simulink model "quadrotor_dynamics_model"  (R2024b)
settings: Solver=VariableStepAuto  StartTime=0.0  FixedStep=0.001  RelTol=1e-3
values from neighbouring files (symbols this model uses):
  a_x_max = 5    [parameters.m]
  a_y_max = 5    [parameters.m]
  a_z_max = 5    [parameters.m]
  angle_max = 0.1745    [parameters.m]
  g = 9.81    [parameters.m]
  Ixx = 5e-3    (= 0.005)    [parameters.m]
  Iyy = 5e-3    (= 0.005)    [parameters.m]
  Izz = 1e-2    (= 0.01)    [parameters.m]
  Jr = 3e-5    (= 3e-05)    [parameters.m]
  K_d_x = 1e-7    (= 1e-07)    [parameters.m]
  K_d_y = 1e-7    (= 1e-07)    [parameters.m]
  K_d_z = 1e-7    (= 1e-07)    [parameters.m]
  Kd = 1e-7    (= 1e-07)    [parameters.m]
  Kd_pqr = [0, 0, 0]    [parameters.m]
  Kd_v = [0, 0, 0]    [parameters.m]
  Ki_pqr = [0.1, 0.1, 0.1]    [parameters.m]
  Ki_v = [0.1, 0.1, 0.1]    [parameters.m]
  Kp_phi = 12    [parameters.m]
  Kp_pqr = [2, 2, 2]    [parameters.m]
  Kp_psi = 10    [parameters.m]
  Kp_theta = 12    [parameters.m]
  Kp_v = [1, 1, 1]    [parameters.m]
  Kp_x = 0.1    [parameters.m]
  Kp_y = 0.1    [parameters.m]
  Kp_z = 0.1    [parameters.m]
  Kt = 3e-6    (= 3e-06)    [parameters.m]
  l = 0.2    [parameters.m]
  m = 0.5    [parameters.m]
  omega_sq_max = 5e+6    (= 5000000)    [parameters.m]
  p_max = 1    [parameters.m]
  q_max = 1    [parameters.m]
  r_max = 1    [parameters.m]
  rpy_dot_in = [0, 0, 0]    [parameters.m]
  rpy_in = [0, 0, 0]    [parameters.m]
  tau_x_max = 0.5    [parameters.m]
  tau_y_max = 0.5    [parameters.m]
  tau_z_max = 0.5    [parameters.m]
  v_x_max = 10    [parameters.m]
  v_y_max = 10    [parameters.m]
  v_z_max = 10    [parameters.m]
  xyz_dot_in = [0, 0, 0]    [parameters.m]
  xyz_in = [0, 0, 0]    [parameters.m]
libraries: slpidlib x6
settings Model: Creator=Ishan  LastModifiedBy=Ishan

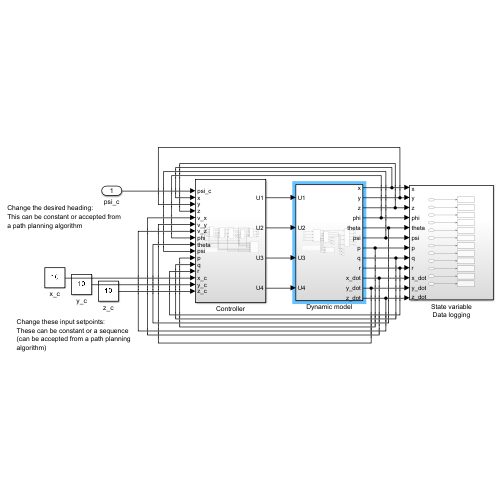
[thumbnail: Simulink's stored preview of the top-level diagram]
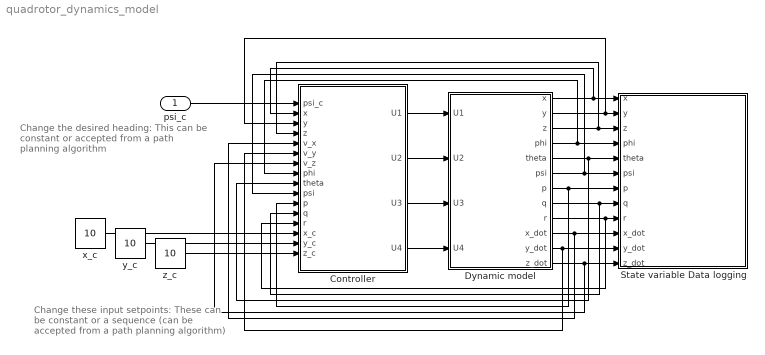
== system quadrotor_dynamics_model ==
  note: Change these input setpoints:
      | These can be constant or a sequence
      | (can be accepted from a path planning
      | algorithm)
  note: Change the desired heading:
      | This can be constant or accepted from
      | a path planning algorithm
  psi_c : Inport
  Controller : Subsystem
  Dynamic model : Subsystem
  State variable Data logging : Subsystem
  x_c : Constant  Value=10
  y_c : Constant  Value=10
  z_c : Constant  Value=10
  wires:
  Controller/4(U4) -> Dynamic model/4(U4)
  Controller/2(U2) -> Dynamic model/2(U2)
  Dynamic model/5(theta) -> Controller/9(theta), State variable Data logging/5(theta)
  Dynamic model/11(y_dot) -> State variable Data logging/11(y_dot), Controller/6(v_y)
  Dynamic model/10(x_dot) -> State variable Data logging/10(x_dot), Controller/5(v_x)
  Dynamic model/8(q) -> Controller/12(q), State variable Data logging/8(q)
  Dynamic model/12(z_dot) -> Controller/7(v_z), State variable Data logging/12(z_dot)
  Dynamic model/4(phi) -> Controller/8(phi), State variable Data logging/4(phi)
  Controller/3(U3) -> Dynamic model/3(U3)
  Dynamic model/3(z) -> Controller/4(z), State variable Data logging/3(z)
  Dynamic model/6(psi) -> State variable Data logging/6(psi), Controller/10(psi)
  Dynamic model/2(y) -> Controller/3(y), State variable Data logging/2(y)
  Dynamic model/1(x) -> Controller/2(x), State variable Data logging/1(x)
  Dynamic model/7(p) -> State variable Data logging/7(p), Controller/11(p)
  Dynamic model/9(r) -> Controller/13(r), State variable Data logging/9(r)
  Controller/1(U1) -> Dynamic model/1(U1)
  x_c/1 -> Controller/14(x_c)
  y_c/1 -> Controller/15(y_c)
  z_c/1 -> Controller/16(z_c)
  psi_c/1 -> Controller/1(psi_c)

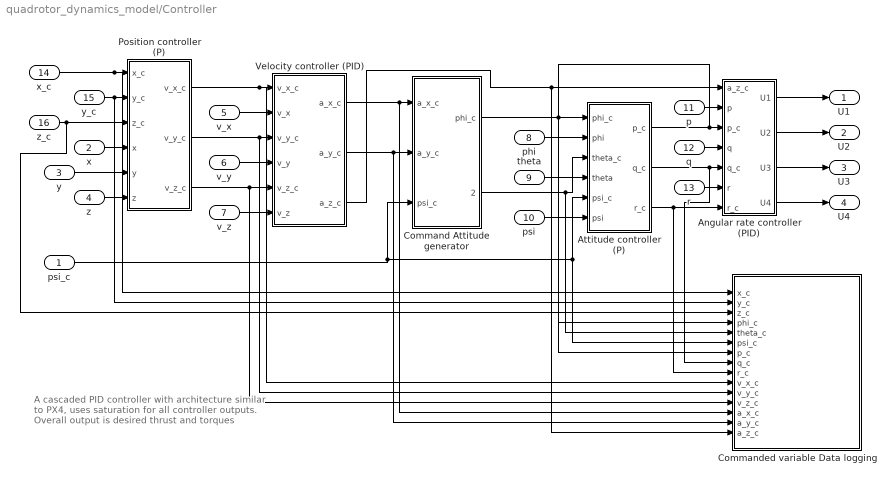
== system quadrotor_dynamics_model/Controller ==
  note: A cascaded PID controller with architecture
      | similar to PX4, uses saturation for all controller
      | outputs. Overall output is desired thrust and
      | torques
  psi_c : Inport
  x : Inport  Port=2
  y : Inport  Port=3
  z : Inport  Port=4
  v_x : Inport  Port=5
  v_y : Inport  Port=6
  v_z : Inport  Port=7
  phi : Inport  Port=8
  theta : Inport  Port=9
  psi : Inport  Port=10
  p : Inport  Port=11
  q : Inport  Port=12
  r : Inport  Port=13
  x_c : Inport  Port=14
  y_c : Inport  Port=15
  z_c : Inport  Port=16
  Angular rate controller (PID) : Subsystem
  Attitude controller (P) : Subsystem
  Command Attitude generator : Subsystem
  Commanded variable Data logging : Subsystem
  Position controller (P) : Subsystem
  Velocity controller (PID) : Subsystem
  U1 : Outport
  U2 : Outport  Port=2
  U3 : Outport  Port=3
  U4 : Outport  Port=4
  wires:
  psi_c/1 -> Command Attitude generator/3(psi_c), Commanded variable Data logging/6(psi_c), Attitude controller (P)/5(psi_c)
  x_c/1 -> Commanded variable Data logging/1(x_c), Position controller (P)/1(x_c)
  y_c/1 -> Commanded variable Data logging/2(y_c), Position controller (P)/2(y_c)
  x/1 -> Position controller (P)/4(x)
  y/1 -> Position controller (P)/5(y)
  z/1 -> Position controller (P)/6(z)
  Position controller (P)/1(v_x_c) -> Commanded variable Data logging/10(v_x_c), Velocity controller (PID)/1(v_x_c)
  Position controller (P)/2(v_y_c) -> Commanded variable Data logging/11(v_y_c), Velocity controller (PID)/3(v_y_c)
  Position controller (P)/3(v_z_c) -> Velocity controller (PID)/5(v_z_c), Commanded variable Data logging/12(v_z_c)
  v_x/1 -> Velocity controller (PID)/2(v_x)
  v_y/1 -> Velocity controller (PID)/4(v_y)
  v_z/1 -> Velocity controller (PID)/6(v_z)
  phi/1 -> Attitude controller (P)/2(phi)
  theta/1 -> Attitude controller (P)/4(theta)
  psi/1 -> Attitude controller (P)/6(psi)
  Attitude controller (P)/1(p_c) -> Commanded variable Data logging/7(p_c), Angular rate controller (PID)/3(p_c)
  Attitude controller (P)/2(q_c) -> Commanded variable Data logging/8(q_c), Angular rate controller (PID)/5(q_c)
  Attitude controller (P)/3(r_c) -> Angular rate controller (PID)/7(r_c), Commanded variable Data logging/9(r_c)
  Velocity controller (PID)/1(a_x_c) -> Commanded variable Data logging/13(a_x_c), Command Attitude generator/1(a_x_c)
  Velocity controller (PID)/2(a_y_c) -> Command Attitude generator/2(a_y_c), Commanded variable Data logging/14(a_y_c)
  Command Attitude generator/1(phi_c) -> Attitude controller (P)/1(phi_c), Commanded variable Data logging/4(phi_c)
  Command Attitude generator/2(theta_c) -> Attitude controller (P)/3(theta_c), Commanded variable Data logging/5(theta_c)
  Velocity controller (PID)/3(a_z_c) -> Angular rate controller (PID)/1(a_z_c), Commanded variable Data logging/15(a_z_c)
  p/1 -> Angular rate controller (PID)/2(p)
  q/1 -> Angular rate controller (PID)/4(q)
  r/1 -> Angular rate controller (PID)/6(r)
  Angular rate controller (PID)/1(U1) -> U1/1
  Angular rate controller (PID)/2(U2) -> U2/1
  Angular rate controller (PID)/3(U3) -> U3/1
  Angular rate controller (PID)/4(U4) -> U4/1
  z_c/1 -> Position controller (P)/3(z_c), Commanded variable Data logging/3(z_c)

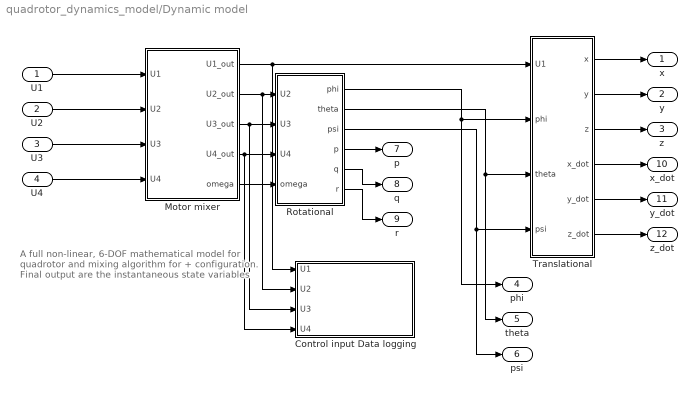
== system quadrotor_dynamics_model/Dynamic model ==
  note: A full non-linear, 6-DOF mathematical model
      | for quadrotor and mixing algorithm for +
      | configuration. Final output are the instantaneous
      | state variables
  U1 : Inport
  U2 : Inport  Port=2
  U3 : Inport  Port=3
  U4 : Inport  Port=4
  Control input Data logging : Subsystem
  Motor mixer : Subsystem
  Rotational : Subsystem
  "Translational " : Subsystem
  x : Outport
  y : Outport  Port=2
  z : Outport  Port=3
  phi : Outport  Port=4
  theta : Outport  Port=5
  psi : Outport  Port=6
  p : Outport  Port=7
  q : Outport  Port=8
  r : Outport  Port=9
  x_dot : Outport  Port=10
  y_dot : Outport  Port=11
  z_dot : Outport  Port=12
  wires:
  "Translational "/1(x) -> x/1
  "Translational "/2(y) -> y/1
  "Translational "/3(z) -> z/1
  Rotational/1(phi) -> phi/1, "Translational "/2(phi)
  U2/1 -> Motor mixer/2(U2)
  U3/1 -> Motor mixer/3(U3)
  U4/1 -> Motor mixer/4(U4)
  "Translational "/4(x_dot) -> x_dot/1
  "Translational "/6(z_dot) -> z_dot/1
  "Translational "/5(y_dot) -> y_dot/1
  Motor mixer/2(U2_out) -> Control input Data logging/2(U2), Rotational/1(U2)
  Motor mixer/3(U3_out) -> Rotational/2(U3), Control input Data logging/3(U3)
  Motor mixer/4(U4_out) -> Control input Data logging/4(U4), Rotational/3(U4)
  Motor mixer/5(omega) -> Rotational/4(omega)
  Rotational/2(theta) -> theta/1, "Translational "/3(theta)
  Rotational/3(psi) -> psi/1, "Translational "/4(psi)
  Rotational/4(p) -> p/1
  Rotational/6(r) -> r/1
  Rotational/5(q) -> q/1
  Motor mixer/1(U1_out) -> Control input Data logging/1(U1), "Translational "/1(U1)
  U1/1 -> Motor mixer/1(U1)

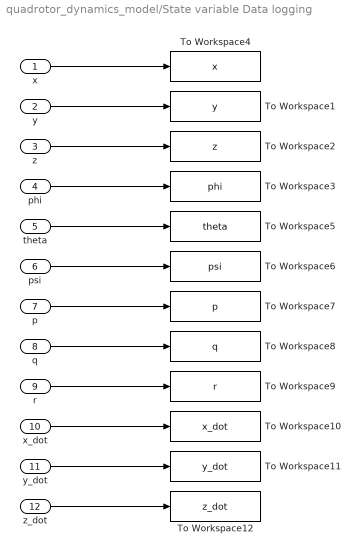
== system quadrotor_dynamics_model/State variable Data logging ==
  x : Inport
  y : Inport  Port=2
  z : Inport  Port=3
  phi : Inport  Port=4
  theta : Inport  Port=5
  psi : Inport  Port=6
  p : Inport  Port=7
  q : Inport  Port=8
  r : Inport  Port=9
  x_dot : Inport  Port=10
  y_dot : Inport  Port=11
  z_dot : Inport  Port=12
  To Workspace1 : ToWorkspace  VariableName=y  SaveFormat=Timeseries  SampleTime=-1
  To Workspace10 : ToWorkspace  VariableName=x_dot  SaveFormat=Timeseries  SampleTime=-1
  To Workspace11 : ToWorkspace  VariableName=y_dot  SaveFormat=Timeseries  SampleTime=-1
  To Workspace12 : ToWorkspace  VariableName=z_dot  SaveFormat=Timeseries  SampleTime=-1
  To Workspace2 : ToWorkspace  VariableName=z  SaveFormat=Timeseries  SampleTime=-1
  To Workspace3 : ToWorkspace  VariableName=phi  SaveFormat=Timeseries  SampleTime=-1
  To Workspace4 : ToWorkspace  VariableName=x  SaveFormat=Timeseries  SampleTime=-1
  To Workspace5 : ToWorkspace  VariableName=theta  SaveFormat=Timeseries  SampleTime=-1
  To Workspace6 : ToWorkspace  VariableName=psi  SaveFormat=Timeseries  SampleTime=-1
  To Workspace7 : ToWorkspace  VariableName=p  SaveFormat=Timeseries  SampleTime=-1
  To Workspace8 : ToWorkspace  VariableName=q  SaveFormat=Timeseries  SampleTime=-1
  To Workspace9 : ToWorkspace  VariableName=r  SaveFormat=Timeseries  SampleTime=-1
  wires:
  x/1 -> To Workspace4/1
  y/1 -> To Workspace1/1
  z/1 -> To Workspace2/1
  phi/1 -> To Workspace3/1
  theta/1 -> To Workspace5/1
  psi/1 -> To Workspace6/1
  p/1 -> To Workspace7/1
  q/1 -> To Workspace8/1
  r/1 -> To Workspace9/1
  x_dot/1 -> To Workspace10/1
  y_dot/1 -> To Workspace11/1
  z_dot/1 -> To Workspace12/1

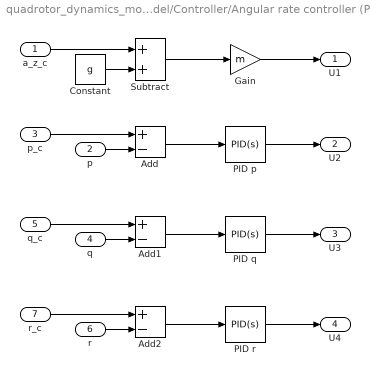
== system quadrotor_dynamics_model/Controller/Angular rate controller (PID) ==
  a_z_c : Inport
  p : Inport  Port=2
  p_c : Inport  Port=3
  q : Inport  Port=4
  q_c : Inport  Port=5
  r : Inport  Port=6
  r_c : Inport  Port=7
  Add : Sum  Inputs=+-
  Add1 : Sum  Inputs=+-
  Add2 : Sum  Inputs=+-
  Constant : Constant  Value=g
  Gain : Gain  Gain=m
  PID p : slpidlib/PID Controller  Controller=PID  Form=Parallel  TimeDomain=Continuous-time  UseExternalTs=off  SampleTime=-1  IntegratorMethod=Forward Euler  FilterMethod=Forward Euler  ControllerParametersSource=internal  P=Kp_pqr(1)  I=Ki_pqr(1)  UseKiTs=off  D=Kd_pqr(1)  UseExternalDerivativeSource=off  N=100000  UseFilter=on  TunerSelectOption=Transfer Function Based (PID Tuner App)  ZeroCross=off  InitialConditionSource=internal  InitialConditionForIntegrator=0  InitialConditionForFilter=0  DifferentiatorICPrevScaledInput=0  ExternalReset=none  TrackingMode=off  Kt=1  LimitOutput=on  SatLimitsSource=internal  UpperSaturationLimit=tau_x_max  LowerSaturationLimit=-tau_x_max  LinearizeAsGain=off  AntiWindupMode=none  Kb=1  LimitIntegrator=off  UpperIntegratorSaturationLimit=inf  LowerIntegratorSaturationLimit=-inf  POutMin=[]  POutMax=[]  IOutMin=[]  IOutMax=[]  DOutMin=[]  DOutMax=[]  NOutMin=[]  NOutMax=[]  SumOutMin=[]  SumOutMax=[]  SaturationOutMin=[]  SaturationOutMax=[]  PParamMin=[]  PParamMax=[]  IParamMin=[]  IParamMax=[]  DParamMin=[]  DParamMax=[]  NParamMin=[]  NParamMax=[]  KbParamMin=[]  KbParamMax=[]  KtParamMin=[]  KtParamMax=[]  KbOutMin=[]  KbOutMax=[]  KtOutMin=[]  KtOutMax=[]  IntegratorOutMin=[]  IntegratorOutMax=[]  FilterOutMin=[]  FilterOutMax=[]  SumI1OutMin=[]  SumI1OutMax=[]  SumI2OutMin=[]  SumI2OutMax=[]  SumI3OutMin=[]  SumI3OutMax=[]  SumI4OutMin=[]  SumI4OutMax=[]  SumDOutMin=[]  SumDOutMax=[]  DifferentiatorOutMin=[]  DifferentiatorOutMax=[]  FilterDiffOutCoefMin=[]  FilterDiffOutCoefMax=[]  ReciprocalOutMin=[]  ReciprocalOutMax=[]  SumDenOutMin=[]  SumDenOutMax=[]  SumNumOutMin=[]  SumNumOutMax=[]  DivideOutMin=[]  DivideOutMax=[]  UdiffTsProdOutMin=[]  UdiffTsProdOutMax=[]  NTsProdOutMin=[]  NTsProdOutMax=[]  UintegralTsProdOutMin=[]  UintegralTsProdOutMax=[]  UngainTsProdOutMin=[]  UngainTsProdOutMax=[]  ClampingZeroOutDataTypeStr=Inherit: Inherit via back propagation  ClampingZeroOutMin=[]  ClampingZeroOutMax=[]  FilterDenConstantOutDataTypeStr=Inherit: Inherit via back propagation  FilterDenConstantOutMin=[]  FilterDenConstantOutMax=[]  PCopyOutDataTypeStr=Inherit: Inherit via back propagation  PCopyOutMin=[]  PCopyOutMax=[]  NCopyOutDataTypeStr=Inherit: Inherit via back propagation  NCopyOutMin=[]  NCopyOutMax=[]  IntegratorContinuousStateAttributes=''  IntegratorStateMustResolveToSignalObject=off  IntegratorRTWStateStorageClass=Auto  FilterContinuousStateAttributes=''  FilterStateMustResolveToSignalObject=off  FilterRTWStateStorageClass=Auto  ParallelPVariant=InternalParameters  IdealPVariant=Disabled  IVariant=InternalParameters  DVariant=InternalParameters  IntegratorVariant=Continuous  SatVariant=Enabled  AWVariant=Passthrough  PCopyVariant=Disabled  TRVariant=Disabled  FdbkBlocksVariant=Forward  IdealPFdbkVariant=Disabled  SatFdbkVariant=Disabled  DerivativeFilterVariant=ContFilter  NVariant=InternalParameters  NCopyVariant=Disabled  FilterICVariant=InternalICsFilter  IntegratorICVariant=InternalICs  ExternalResetVariant=Disabled  TRSumVariant=Passthrough  SumFdbkVariant=Disabled  SumVariant=Sum_PID  TsampFilterVariant=InternalTs  TsampNgainVariant=Passthrough  TsampIntegralVariant=Disabled_SignalSpec  ExternalSaturationOutDataTypeStr=Inherit: Same as second input  DerivativeSourceVariant=ErrorSignal  PreIntVariant=InternalPreInt
  PID q : slpidlib/PID Controller  Controller=PID  Form=Parallel  TimeDomain=Continuous-time  UseExternalTs=off  SampleTime=-1  IntegratorMethod=Forward Euler  FilterMethod=Forward Euler  ControllerParametersSource=internal  P=Kp_pqr(2)  I=Ki_pqr(2)  UseKiTs=off  D=Kd_pqr(2)  UseExternalDerivativeSource=off  N=100000  UseFilter=on  TunerSelectOption=Transfer Function Based (PID Tuner App)  ZeroCross=off  InitialConditionSource=internal  InitialConditionForIntegrator=0  InitialConditionForFilter=0  DifferentiatorICPrevScaledInput=0  ExternalReset=none  TrackingMode=off  Kt=1  LimitOutput=on  SatLimitsSource=internal  UpperSaturationLimit=tau_y_max  LowerSaturationLimit=-tau_y_max  LinearizeAsGain=off  AntiWindupMode=none  Kb=1  LimitIntegrator=off  UpperIntegratorSaturationLimit=inf  LowerIntegratorSaturationLimit=-inf  POutMin=[]  POutMax=[]  IOutMin=[]  IOutMax=[]  DOutMin=[]  DOutMax=[]  NOutMin=[]  NOutMax=[]  SumOutMin=[]  SumOutMax=[]  SaturationOutMin=[]  SaturationOutMax=[]  PParamMin=[]  PParamMax=[]  IParamMin=[]  IParamMax=[]  DParamMin=[]  DParamMax=[]  NParamMin=[]  NParamMax=[]  KbParamMin=[]  KbParamMax=[]  KtParamMin=[]  KtParamMax=[]  KbOutMin=[]  KbOutMax=[]  KtOutMin=[]  KtOutMax=[]  IntegratorOutMin=[]  IntegratorOutMax=[]  FilterOutMin=[]  FilterOutMax=[]  SumI1OutMin=[]  SumI1OutMax=[]  SumI2OutMin=[]  SumI2OutMax=[]  SumI3OutMin=[]  SumI3OutMax=[]  SumI4OutMin=[]  SumI4OutMax=[]  SumDOutMin=[]  SumDOutMax=[]  DifferentiatorOutMin=[]  DifferentiatorOutMax=[]  FilterDiffOutCoefMin=[]  FilterDiffOutCoefMax=[]  ReciprocalOutMin=[]  ReciprocalOutMax=[]  SumDenOutMin=[]  SumDenOutMax=[]  SumNumOutMin=[]  SumNumOutMax=[]  DivideOutMin=[]  DivideOutMax=[]  UdiffTsProdOutMin=[]  UdiffTsProdOutMax=[]  NTsProdOutMin=[]  NTsProdOutMax=[]  UintegralTsProdOutMin=[]  UintegralTsProdOutMax=[]  UngainTsProdOutMin=[]  UngainTsProdOutMax=[]  ClampingZeroOutDataTypeStr=Inherit: Inherit via back propagation  ClampingZeroOutMin=[]  ClampingZeroOutMax=[]  FilterDenConstantOutDataTypeStr=Inherit: Inherit via back propagation  FilterDenConstantOutMin=[]  FilterDenConstantOutMax=[]  PCopyOutDataTypeStr=Inherit: Inherit via back propagation  PCopyOutMin=[]  PCopyOutMax=[]  NCopyOutDataTypeStr=Inherit: Inherit via back propagation  NCopyOutMin=[]  NCopyOutMax=[]  IntegratorContinuousStateAttributes=''  IntegratorStateMustResolveToSignalObject=off  IntegratorRTWStateStorageClass=Auto  FilterContinuousStateAttributes=''  FilterStateMustResolveToSignalObject=off  FilterRTWStateStorageClass=Auto  ParallelPVariant=InternalParameters  IdealPVariant=Disabled  IVariant=InternalParameters  DVariant=InternalParameters  IntegratorVariant=Continuous  SatVariant=Enabled  AWVariant=Passthrough  PCopyVariant=Disabled  TRVariant=Disabled  FdbkBlocksVariant=Forward  IdealPFdbkVariant=Disabled  SatFdbkVariant=Disabled  DerivativeFilterVariant=ContFilter  NVariant=InternalParameters  NCopyVariant=Disabled  FilterICVariant=InternalICsFilter  IntegratorICVariant=InternalICs  ExternalResetVariant=Disabled  TRSumVariant=Passthrough  SumFdbkVariant=Disabled  SumVariant=Sum_PID  TsampFilterVariant=InternalTs  TsampNgainVariant=Passthrough  TsampIntegralVariant=Disabled_SignalSpec  ExternalSaturationOutDataTypeStr=Inherit: Same as second input  DerivativeSourceVariant=ErrorSignal  PreIntVariant=InternalPreInt
  PID r : slpidlib/PID Controller  Controller=PID  Form=Parallel  TimeDomain=Continuous-time  UseExternalTs=off  SampleTime=-1  IntegratorMethod=Forward Euler  FilterMethod=Forward Euler  ControllerParametersSource=internal  P=Kp_pqr(3)  I=Ki_pqr(3)  UseKiTs=off  D=Kd_pqr(3)  UseExternalDerivativeSource=off  N=100000  UseFilter=on  TunerSelectOption=Transfer Function Based (PID Tuner App)  ZeroCross=off  InitialConditionSource=internal  InitialConditionForIntegrator=0  InitialConditionForFilter=0  DifferentiatorICPrevScaledInput=0  ExternalReset=none  TrackingMode=off  Kt=1  LimitOutput=on  SatLimitsSource=internal  UpperSaturationLimit=tau_z_max  LowerSaturationLimit=-tau_z_max  LinearizeAsGain=off  AntiWindupMode=none  Kb=1  LimitIntegrator=off  UpperIntegratorSaturationLimit=inf  LowerIntegratorSaturationLimit=-inf  POutMin=[]  POutMax=[]  IOutMin=[]  IOutMax=[]  DOutMin=[]  DOutMax=[]  NOutMin=[]  NOutMax=[]  SumOutMin=[]  SumOutMax=[]  SaturationOutMin=[]  SaturationOutMax=[]  PParamMin=[]  PParamMax=[]  IParamMin=[]  IParamMax=[]  DParamMin=[]  DParamMax=[]  NParamMin=[]  NParamMax=[]  KbParamMin=[]  KbParamMax=[]  KtParamMin=[]  KtParamMax=[]  KbOutMin=[]  KbOutMax=[]  KtOutMin=[]  KtOutMax=[]  IntegratorOutMin=[]  IntegratorOutMax=[]  FilterOutMin=[]  FilterOutMax=[]  SumI1OutMin=[]  SumI1OutMax=[]  SumI2OutMin=[]  SumI2OutMax=[]  SumI3OutMin=[]  SumI3OutMax=[]  SumI4OutMin=[]  SumI4OutMax=[]  SumDOutMin=[]  SumDOutMax=[]  DifferentiatorOutMin=[]  DifferentiatorOutMax=[]  FilterDiffOutCoefMin=[]  FilterDiffOutCoefMax=[]  ReciprocalOutMin=[]  ReciprocalOutMax=[]  SumDenOutMin=[]  SumDenOutMax=[]  SumNumOutMin=[]  SumNumOutMax=[]  DivideOutMin=[]  DivideOutMax=[]  UdiffTsProdOutMin=[]  UdiffTsProdOutMax=[]  NTsProdOutMin=[]  NTsProdOutMax=[]  UintegralTsProdOutMin=[]  UintegralTsProdOutMax=[]  UngainTsProdOutMin=[]  UngainTsProdOutMax=[]  ClampingZeroOutDataTypeStr=Inherit: Inherit via back propagation  ClampingZeroOutMin=[]  ClampingZeroOutMax=[]  FilterDenConstantOutDataTypeStr=Inherit: Inherit via back propagation  FilterDenConstantOutMin=[]  FilterDenConstantOutMax=[]  PCopyOutDataTypeStr=Inherit: Inherit via back propagation  PCopyOutMin=[]  PCopyOutMax=[]  NCopyOutDataTypeStr=Inherit: Inherit via back propagation  NCopyOutMin=[]  NCopyOutMax=[]  IntegratorContinuousStateAttributes=''  IntegratorStateMustResolveToSignalObject=off  IntegratorRTWStateStorageClass=Auto  FilterContinuousStateAttributes=''  FilterStateMustResolveToSignalObject=off  FilterRTWStateStorageClass=Auto  ParallelPVariant=InternalParameters  IdealPVariant=Disabled  IVariant=InternalParameters  DVariant=InternalParameters  IntegratorVariant=Continuous  SatVariant=Enabled  AWVariant=Passthrough  PCopyVariant=Disabled  TRVariant=Disabled  FdbkBlocksVariant=Forward  IdealPFdbkVariant=Disabled  SatFdbkVariant=Disabled  DerivativeFilterVariant=ContFilter  NVariant=InternalParameters  NCopyVariant=Disabled  FilterICVariant=InternalICsFilter  IntegratorICVariant=InternalICs  ExternalResetVariant=Disabled  TRSumVariant=Passthrough  SumFdbkVariant=Disabled  SumVariant=Sum_PID  TsampFilterVariant=InternalTs  TsampNgainVariant=Passthrough  TsampIntegralVariant=Disabled_SignalSpec  ExternalSaturationOutDataTypeStr=Inherit: Same as second input  DerivativeSourceVariant=ErrorSignal  PreIntVariant=InternalPreInt
  Subtract : Sum
  U1 : Outport
  U2 : Outport  Port=2
  U3 : Outport  Port=3
  U4 : Outport  Port=4
  wires:
  Add/1 -> PID p/1
  PID p/1 -> U2/1
  PID q/1 -> U3/1
  Add1/1 -> PID q/1
  PID r/1 -> U4/1
  Add2/1 -> PID r/1
  p_c/1 -> Add/1
  p/1 -> Add/2
  q_c/1 -> Add1/1
  q/1 -> Add1/2
  r_c/1 -> Add2/1
  r/1 -> Add2/2
  a_z_c/1 -> Subtract/1
  Constant/1 -> Subtract/2
  Subtract/1 -> Gain/1
  Gain/1 -> U1/1

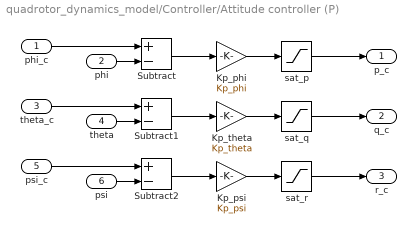
== system quadrotor_dynamics_model/Controller/Attitude controller (P) ==
  phi_c : Inport
  phi : Inport  Port=2
  theta_c : Inport  Port=3
  theta : Inport  Port=4
  psi_c : Inport  Port=5
  psi : Inport  Port=6
  Kp_phi : Gain  Gain=Kp_phi
  Kp_psi : Gain  Gain=Kp_psi
  Kp_theta : Gain  Gain=Kp_theta
  Subtract : Sum  Inputs=+-
  Subtract1 : Sum  Inputs=+-
  Subtract2 : Sum  Inputs=+-
  sat_p : Saturate  UpperLimit=p_max  LowerLimit=-p_max  LinearizeAsGain=off  ZeroCross=off
  sat_q : Saturate  UpperLimit=q_max  LowerLimit=-q_max  LinearizeAsGain=off  ZeroCross=off
  sat_r : Saturate  UpperLimit=r_max  LowerLimit=-r_max  LinearizeAsGain=off  ZeroCross=off
  p_c : Outport
  q_c : Outport  Port=2
  r_c : Outport  Port=3
  wires:
  Kp_phi/1 -> sat_p/1
  phi/1 -> Subtract/2
  phi_c/1 -> Subtract/1
  Subtract/1 -> Kp_phi/1
  theta_c/1 -> Subtract1/1
  theta/1 -> Subtract1/2
  Subtract1/1 -> Kp_theta/1
  Kp_theta/1 -> sat_q/1
  psi/1 -> Subtract2/2
  psi_c/1 -> Subtract2/1
  Subtract2/1 -> Kp_psi/1
  Kp_psi/1 -> sat_r/1
  sat_p/1 -> p_c/1
  sat_q/1 -> q_c/1
  sat_r/1 -> r_c/1

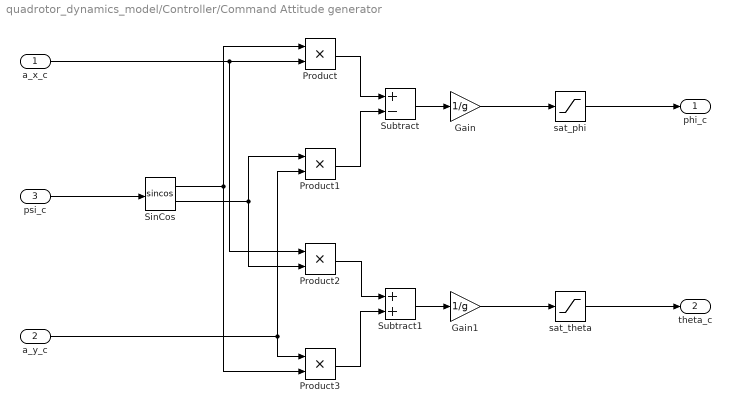
== system quadrotor_dynamics_model/Controller/Command Attitude generator ==
  a_x_c : Inport
  a_y_c : Inport  Port=2
  psi_c : Inport  Port=3
  Gain : Gain  Gain=1/g
  Gain1 : Gain  Gain=1/g
  Product{,1..3} (4 alike) : Product
  SinCos : Trigonometry  Operator=sincos
  Subtract : Sum  Inputs=+-
  Subtract1 : Sum
  sat_phi : Saturate  UpperLimit=angle_max  LowerLimit=-angle_max  LinearizeAsGain=off  ZeroCross=off
  sat_theta : Saturate  UpperLimit=angle_max  LowerLimit=-angle_max  LinearizeAsGain=off  ZeroCross=off
  phi_c : Outport
  theta_c : Outport  Port=2
  wires:
  sat_theta/1 -> theta_c/1
  Gain1/1 -> sat_theta/1
  sat_phi/1 -> phi_c/1
  Subtract1/1 -> Gain1/1
  psi_c/1 -> SinCos/1
  Product1/1 -> Subtract/2
  Gain/1 -> sat_phi/1
  Product3/1 -> Subtract1/2
  SinCos/2 -> Product2/2, Product1/1
  Subtract/1 -> Gain/1
  a_x_c/1 -> Product/2, Product2/1
  Product/1 -> Subtract/1
  Product2/1 -> Subtract1/1
  SinCos/1 -> Product3/2, Product/1
  a_y_c/1 -> Product3/1, Product1/2

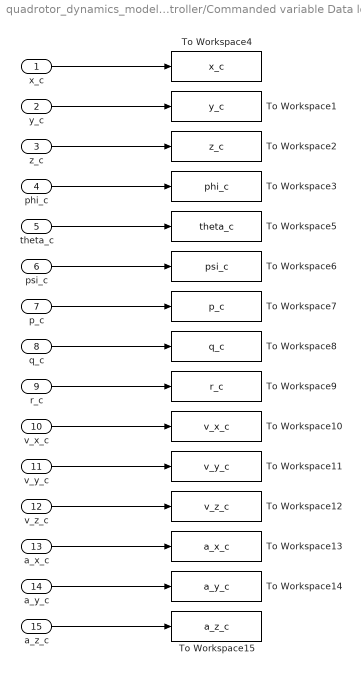
== system quadrotor_dynamics_model/Controller/Commanded variable Data logging ==
  x_c : Inport
  y_c : Inport  Port=2
  z_c : Inport  Port=3
  phi_c : Inport  Port=4
  theta_c : Inport  Port=5
  psi_c : Inport  Port=6
  p_c : Inport  Port=7
  q_c : Inport  Port=8
  r_c : Inport  Port=9
  v_x_c : Inport  Port=10
  v_y_c : Inport  Port=11
  v_z_c : Inport  Port=12
  a_x_c : Inport  Port=13
  a_y_c : Inport  Port=14
  a_z_c : Inport  Port=15
  To Workspace1 : ToWorkspace  VariableName=y_c  SaveFormat=Timeseries  SampleTime=-1
  To Workspace10 : ToWorkspace  VariableName=v_x_c  SaveFormat=Timeseries  SampleTime=-1
  To Workspace11 : ToWorkspace  VariableName=v_y_c  SaveFormat=Timeseries  SampleTime=-1
  To Workspace12 : ToWorkspace  VariableName=v_z_c  SaveFormat=Timeseries  SampleTime=-1
  To Workspace13 : ToWorkspace  VariableName=a_x_c  SaveFormat=Timeseries  SampleTime=-1
  To Workspace14 : ToWorkspace  VariableName=a_y_c  SaveFormat=Timeseries  SampleTime=-1
  To Workspace15 : ToWorkspace  VariableName=a_z_c  SaveFormat=Timeseries  SampleTime=-1
  To Workspace2 : ToWorkspace  VariableName=z_c  SaveFormat=Timeseries  SampleTime=-1
  To Workspace3 : ToWorkspace  VariableName=phi_c  SaveFormat=Timeseries  SampleTime=-1
  To Workspace4 : ToWorkspace  VariableName=x_c  SaveFormat=Timeseries  SampleTime=-1
  To Workspace5 : ToWorkspace  VariableName=theta_c  SaveFormat=Timeseries  SampleTime=-1
  To Workspace6 : ToWorkspace  VariableName=psi_c  SaveFormat=Timeseries  SampleTime=-1
  To Workspace7 : ToWorkspace  VariableName=p_c  SaveFormat=Timeseries  SampleTime=-1
  To Workspace8 : ToWorkspace  VariableName=q_c  SaveFormat=Timeseries  SampleTime=-1
  To Workspace9 : ToWorkspace  VariableName=r_c  SaveFormat=Timeseries  SampleTime=-1
  wires:
  x_c/1 -> To Workspace4/1
  y_c/1 -> To Workspace1/1
  z_c/1 -> To Workspace2/1
  phi_c/1 -> To Workspace3/1
  theta_c/1 -> To Workspace5/1
  psi_c/1 -> To Workspace6/1
  p_c/1 -> To Workspace7/1
  q_c/1 -> To Workspace8/1
  r_c/1 -> To Workspace9/1
  v_x_c/1 -> To Workspace10/1
  v_y_c/1 -> To Workspace11/1
  v_z_c/1 -> To Workspace12/1
  a_z_c/1 -> To Workspace15/1
  a_y_c/1 -> To Workspace14/1
  a_x_c/1 -> To Workspace13/1

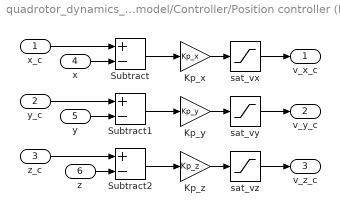
== system quadrotor_dynamics_model/Controller/Position controller (P) ==
  x_c : Inport
  y_c : Inport  Port=2
  z_c : Inport  Port=3
  x : Inport  Port=4
  y : Inport  Port=5
  z : Inport  Port=6
  Kp_x : Gain  Gain=Kp_x
  Kp_y : Gain  Gain=Kp_y
  Kp_z : Gain  Gain=Kp_z
  Subtract : Sum  Inputs=+-
  Subtract1 : Sum  Inputs=+-
  Subtract2 : Sum  Inputs=+-
  sat_vx : Saturate  UpperLimit=v_x_max  LowerLimit=-v_x_max
  sat_vy : Saturate  UpperLimit=v_y_max  LowerLimit=-v_y_max
  sat_vz : Saturate  UpperLimit=v_z_max  LowerLimit=-v_z_max
  v_x_c : Outport
  v_y_c : Outport  Port=2
  v_z_c : Outport  Port=3
  wires:
  z_c/1 -> Subtract2/1
  Subtract/1 -> Kp_x/1
  Subtract2/1 -> Kp_z/1
  x_c/1 -> Subtract/1
  Subtract1/1 -> Kp_y/1
  y/1 -> Subtract1/2
  Kp_y/1 -> sat_vy/1
  Kp_z/1 -> sat_vz/1
  Kp_x/1 -> sat_vx/1
  x/1 -> Subtract/2
  y_c/1 -> Subtract1/1
  z/1 -> Subtract2/2
  sat_vx/1 -> v_x_c/1
  sat_vy/1 -> v_y_c/1
  sat_vz/1 -> v_z_c/1

== system quadrotor_dynamics_model/Controller/Velocity controller (PID) ==
  v_x_c : Inport
  v_x : Inport  Port=2
  v_y_c : Inport  Port=3
  v_y : Inport  Port=4
  v_z_c : Inport  Port=5
  v_z : Inport  Port=6
  PID v_x : slpidlib/PID Controller  Controller=PID  Form=Parallel  TimeDomain=Continuous-time  UseExternalTs=off  SampleTime=-1  IntegratorMethod=Forward Euler  FilterMethod=Forward Euler  ControllerParametersSource=internal  P=Kp_v(1)  I=Ki_v(1)  UseKiTs=off  D=Kd_v(1)  UseExternalDerivativeSource=off  N=1000000  UseFilter=on  TunerSelectOption=Transfer Function Based (PID Tuner App)  ZeroCross=off  InitialConditionSource=internal  InitialConditionForIntegrator=0  InitialConditionForFilter=0  DifferentiatorICPrevScaledInput=0  ExternalReset=none  TrackingMode=off  Kt=1  LimitOutput=on  SatLimitsSource=internal  UpperSaturationLimit=a_x_max  LowerSaturationLimit=-a_x_max  LinearizeAsGain=off  AntiWindupMode=none  Kb=1  LimitIntegrator=off  UpperIntegratorSaturationLimit=inf  LowerIntegratorSaturationLimit=-inf  POutMin=[]  POutMax=[]  IOutMin=[]  IOutMax=[]  DOutMin=[]  DOutMax=[]  NOutMin=[]  NOutMax=[]  SumOutMin=[]  SumOutMax=[]  SaturationOutMin=[]  SaturationOutMax=[]  PParamMin=[]  PParamMax=[]  IParamMin=[]  IParamMax=[]  DParamMin=[]  DParamMax=[]  NParamMin=[]  NParamMax=[]  KbParamMin=[]  KbParamMax=[]  KtParamMin=[]  KtParamMax=[]  KbOutMin=[]  KbOutMax=[]  KtOutMin=[]  KtOutMax=[]  IntegratorOutMin=[]  IntegratorOutMax=[]  FilterOutMin=[]  FilterOutMax=[]  SumI1OutMin=[]  SumI1OutMax=[]  SumI2OutMin=[]  SumI2OutMax=[]  SumI3OutMin=[]  SumI3OutMax=[]  SumI4OutMin=[]  SumI4OutMax=[]  SumDOutMin=[]  SumDOutMax=[]  DifferentiatorOutMin=[]  DifferentiatorOutMax=[]  FilterDiffOutCoefMin=[]  FilterDiffOutCoefMax=[]  ReciprocalOutMin=[]  ReciprocalOutMax=[]  SumDenOutMin=[]  SumDenOutMax=[]  SumNumOutMin=[]  SumNumOutMax=[]  DivideOutMin=[]  DivideOutMax=[]  UdiffTsProdOutMin=[]  UdiffTsProdOutMax=[]  NTsProdOutMin=[]  NTsProdOutMax=[]  UintegralTsProdOutMin=[]  UintegralTsProdOutMax=[]  UngainTsProdOutMin=[]  UngainTsProdOutMax=[]  ClampingZeroOutDataTypeStr=Inherit: Inherit via back propagation  ClampingZeroOutMin=[]  ClampingZeroOutMax=[]  FilterDenConstantOutDataTypeStr=Inherit: Inherit via back propagation  FilterDenConstantOutMin=[]  FilterDenConstantOutMax=[]  PCopyOutDataTypeStr=Inherit: Inherit via back propagation  PCopyOutMin=[]  PCopyOutMax=[]  NCopyOutDataTypeStr=Inherit: Inherit via back propagation  NCopyOutMin=[]  NCopyOutMax=[]  IntegratorContinuousStateAttributes=''  IntegratorStateMustResolveToSignalObject=off  IntegratorRTWStateStorageClass=Auto  FilterContinuousStateAttributes=''  FilterStateMustResolveToSignalObject=off  FilterRTWStateStorageClass=Auto  ParallelPVariant=InternalParameters  IdealPVariant=Disabled  IVariant=InternalParameters  DVariant=InternalParameters  IntegratorVariant=Continuous  SatVariant=Enabled  AWVariant=Passthrough  PCopyVariant=Disabled  TRVariant=Disabled  FdbkBlocksVariant=Forward  IdealPFdbkVariant=Disabled  SatFdbkVariant=Disabled  DerivativeFilterVariant=ContFilter  NVariant=InternalParameters  NCopyVariant=Disabled  FilterICVariant=InternalICsFilter  IntegratorICVariant=InternalICs  ExternalResetVariant=Disabled  TRSumVariant=Passthrough  SumFdbkVariant=Disabled  SumVariant=Sum_PID  TsampFilterVariant=InternalTs  TsampNgainVariant=Passthrough  TsampIntegralVariant=Disabled_SignalSpec  ExternalSaturationOutDataTypeStr=Inherit: Same as second input  DerivativeSourceVariant=ErrorSignal  PreIntVariant=InternalPreInt
  PID v_y : slpidlib/PID Controller  Controller=PID  Form=Parallel  TimeDomain=Continuous-time  UseExternalTs=off  SampleTime=-1  IntegratorMethod=Forward Euler  FilterMethod=Forward Euler  ControllerParametersSource=internal  P=Kp_v(2)  I=Ki_v(2)  UseKiTs=off  D=Kd_v(2)  UseExternalDerivativeSource=off  N=1000000  UseFilter=on  TunerSelectOption=Transfer Function Based (PID Tuner App)  ZeroCross=off  InitialConditionSource=internal  InitialConditionForIntegrator=0  InitialConditionForFilter=0  DifferentiatorICPrevScaledInput=0  ExternalReset=none  TrackingMode=off  Kt=1  LimitOutput=on  SatLimitsSource=internal  UpperSaturationLimit=a_y_max  LowerSaturationLimit=-a_y_max  LinearizeAsGain=on  AntiWindupMode=none  Kb=1  LimitIntegrator=off  UpperIntegratorSaturationLimit=inf  LowerIntegratorSaturationLimit=-inf  POutMin=[]  POutMax=[]  IOutMin=[]  IOutMax=[]  DOutMin=[]  DOutMax=[]  NOutMin=[]  NOutMax=[]  SumOutMin=[]  SumOutMax=[]  SaturationOutMin=[]  SaturationOutMax=[]  PParamMin=[]  PParamMax=[]  IParamMin=[]  IParamMax=[]  DParamMin=[]  DParamMax=[]  NParamMin=[]  NParamMax=[]  KbParamMin=[]  KbParamMax=[]  KtParamMin=[]  KtParamMax=[]  KbOutMin=[]  KbOutMax=[]  KtOutMin=[]  KtOutMax=[]  IntegratorOutMin=[]  IntegratorOutMax=[]  FilterOutMin=[]  FilterOutMax=[]  SumI1OutMin=[]  SumI1OutMax=[]  SumI2OutMin=[]  SumI2OutMax=[]  SumI3OutMin=[]  SumI3OutMax=[]  SumI4OutMin=[]  SumI4OutMax=[]  SumDOutMin=[]  SumDOutMax=[]  DifferentiatorOutMin=[]  DifferentiatorOutMax=[]  FilterDiffOutCoefMin=[]  FilterDiffOutCoefMax=[]  ReciprocalOutMin=[]  ReciprocalOutMax=[]  SumDenOutMin=[]  SumDenOutMax=[]  SumNumOutMin=[]  SumNumOutMax=[]  DivideOutMin=[]  DivideOutMax=[]  UdiffTsProdOutMin=[]  UdiffTsProdOutMax=[]  NTsProdOutMin=[]  NTsProdOutMax=[]  UintegralTsProdOutMin=[]  UintegralTsProdOutMax=[]  UngainTsProdOutMin=[]  UngainTsProdOutMax=[]  ClampingZeroOutDataTypeStr=Inherit: Inherit via back propagation  ClampingZeroOutMin=[]  ClampingZeroOutMax=[]  FilterDenConstantOutDataTypeStr=Inherit: Inherit via back propagation  FilterDenConstantOutMin=[]  FilterDenConstantOutMax=[]  PCopyOutDataTypeStr=Inherit: Inherit via back propagation  PCopyOutMin=[]  PCopyOutMax=[]  NCopyOutDataTypeStr=Inherit: Inherit via back propagation  NCopyOutMin=[]  NCopyOutMax=[]  IntegratorContinuousStateAttributes=''  IntegratorStateMustResolveToSignalObject=off  IntegratorRTWStateStorageClass=Auto  FilterContinuousStateAttributes=''  FilterStateMustResolveToSignalObject=off  FilterRTWStateStorageClass=Auto  ParallelPVariant=InternalParameters  IdealPVariant=Disabled  IVariant=InternalParameters  DVariant=InternalParameters  IntegratorVariant=Continuous  SatVariant=Enabled  AWVariant=Passthrough  PCopyVariant=Disabled  TRVariant=Disabled  FdbkBlocksVariant=Forward  IdealPFdbkVariant=Disabled  SatFdbkVariant=Disabled  DerivativeFilterVariant=ContFilter  NVariant=InternalParameters  NCopyVariant=Disabled  FilterICVariant=InternalICsFilter  IntegratorICVariant=InternalICs  ExternalResetVariant=Disabled  TRSumVariant=Passthrough  SumFdbkVariant=Disabled  SumVariant=Sum_PID  TsampFilterVariant=InternalTs  TsampNgainVariant=Passthrough  TsampIntegralVariant=Disabled_SignalSpec  ExternalSaturationOutDataTypeStr=Inherit: Same as second input  DerivativeSourceVariant=ErrorSignal  PreIntVariant=InternalPreInt
  PID v_z : slpidlib/PID Controller  Controller=PID  Form=Parallel  TimeDomain=Continuous-time  UseExternalTs=off  SampleTime=-1  IntegratorMethod=Forward Euler  FilterMethod=Forward Euler  ControllerParametersSource=internal  P=Kp_v(3)  I=Ki_v(3)  UseKiTs=off  D=Kd_v(3)  UseExternalDerivativeSource=off  N=1000000  UseFilter=on  TunerSelectOption=Transfer Function Based (PID Tuner App)  ZeroCross=off  InitialConditionSource=internal  InitialConditionForIntegrator=0  InitialConditionForFilter=0  DifferentiatorICPrevScaledInput=0  ExternalReset=none  TrackingMode=off  Kt=1  LimitOutput=on  SatLimitsSource=internal  UpperSaturationLimit=a_z_max  LowerSaturationLimit=-a_z_max  LinearizeAsGain=on  AntiWindupMode=none  Kb=1  LimitIntegrator=off  UpperIntegratorSaturationLimit=inf  LowerIntegratorSaturationLimit=-inf  POutMin=[]  POutMax=[]  IOutMin=[]  IOutMax=[]  DOutMin=[]  DOutMax=[]  NOutMin=[]  NOutMax=[]  SumOutMin=[]  SumOutMax=[]  SaturationOutMin=[]  SaturationOutMax=[]  PParamMin=[]  PParamMax=[]  IParamMin=[]  IParamMax=[]  DParamMin=[]  DParamMax=[]  NParamMin=[]  NParamMax=[]  KbParamMin=[]  KbParamMax=[]  KtParamMin=[]  KtParamMax=[]  KbOutMin=[]  KbOutMax=[]  KtOutMin=[]  KtOutMax=[]  IntegratorOutMin=[]  IntegratorOutMax=[]  FilterOutMin=[]  FilterOutMax=[]  SumI1OutMin=[]  SumI1OutMax=[]  SumI2OutMin=[]  SumI2OutMax=[]  SumI3OutMin=[]  SumI3OutMax=[]  SumI4OutMin=[]  SumI4OutMax=[]  SumDOutMin=[]  SumDOutMax=[]  DifferentiatorOutMin=[]  DifferentiatorOutMax=[]  FilterDiffOutCoefMin=[]  FilterDiffOutCoefMax=[]  ReciprocalOutMin=[]  ReciprocalOutMax=[]  SumDenOutMin=[]  SumDenOutMax=[]  SumNumOutMin=[]  SumNumOutMax=[]  DivideOutMin=[]  DivideOutMax=[]  UdiffTsProdOutMin=[]  UdiffTsProdOutMax=[]  NTsProdOutMin=[]  NTsProdOutMax=[]  UintegralTsProdOutMin=[]  UintegralTsProdOutMax=[]  UngainTsProdOutMin=[]  UngainTsProdOutMax=[]  ClampingZeroOutDataTypeStr=Inherit: Inherit via back propagation  ClampingZeroOutMin=[]  ClampingZeroOutMax=[]  FilterDenConstantOutDataTypeStr=Inherit: Inherit via back propagation  FilterDenConstantOutMin=[]  FilterDenConstantOutMax=[]  PCopyOutDataTypeStr=Inherit: Inherit via back propagation  PCopyOutMin=[]  PCopyOutMax=[]  NCopyOutDataTypeStr=Inherit: Inherit via back propagation  NCopyOutMin=[]  NCopyOutMax=[]  IntegratorContinuousStateAttributes=''  IntegratorStateMustResolveToSignalObject=off  IntegratorRTWStateStorageClass=Auto  FilterContinuousStateAttributes=''  FilterStateMustResolveToSignalObject=off  FilterRTWStateStorageClass=Auto  ParallelPVariant=InternalParameters  IdealPVariant=Disabled  IVariant=InternalParameters  DVariant=InternalParameters  IntegratorVariant=Continuous  SatVariant=Enabled  AWVariant=Passthrough  PCopyVariant=Disabled  TRVariant=Disabled  FdbkBlocksVariant=Forward  IdealPFdbkVariant=Disabled  SatFdbkVariant=Disabled  DerivativeFilterVariant=ContFilter  NVariant=InternalParameters  NCopyVariant=Disabled  FilterICVariant=InternalICsFilter  IntegratorICVariant=InternalICs  ExternalResetVariant=Disabled  TRSumVariant=Passthrough  SumFdbkVariant=Disabled  SumVariant=Sum_PID  TsampFilterVariant=InternalTs  TsampNgainVariant=Passthrough  TsampIntegralVariant=Disabled_SignalSpec  ExternalSaturationOutDataTypeStr=Inherit: Same as second input  DerivativeSourceVariant=ErrorSignal  PreIntVariant=InternalPreInt
  Subtract : Sum  Inputs=+-
  Subtract1 : Sum  Inputs=+-
  Subtract2 : Sum  Inputs=+-
  a_x_c : Outport
  a_y_c : Outport  Port=2
  a_z_c : Outport  Port=3
  wires:
  v_x_c/1 -> Subtract/1
  v_x/1 -> Subtract/2
  Subtract/1 -> PID v_x/1
  PID v_x/1 -> a_x_c/1
  Subtract1/1 -> PID v_y/1
  v_y_c/1 -> Subtract1/1
  PID v_y/1 -> a_y_c/1
  v_y/1 -> Subtract1/2
  Subtract2/1 -> PID v_z/1
  v_z_c/1 -> Subtract2/1
  PID v_z/1 -> a_z_c/1
  v_z/1 -> Subtract2/2

== system quadrotor_dynamics_model/Dynamic model/Control input Data logging ==
  U1 : Inport
  U2 : Inport  Port=2
  U3 : Inport  Port=3
  U4 : Inport  Port=4
  To Workspace1 : ToWorkspace  VariableName=U2  SaveFormat=Timeseries  SampleTime=-1
  To Workspace2 : ToWorkspace  VariableName=U3  SaveFormat=Timeseries  SampleTime=-1
  To Workspace3 : ToWorkspace  VariableName=U4  SaveFormat=Timeseries  SampleTime=-1
  To Workspace4 : ToWorkspace  VariableName=U1  SaveFormat=Timeseries  SampleTime=-1
  wires:
  U1/1 -> To Workspace4/1
  U2/1 -> To Workspace1/1
  U3/1 -> To Workspace2/1
  U4/1 -> To Workspace3/1

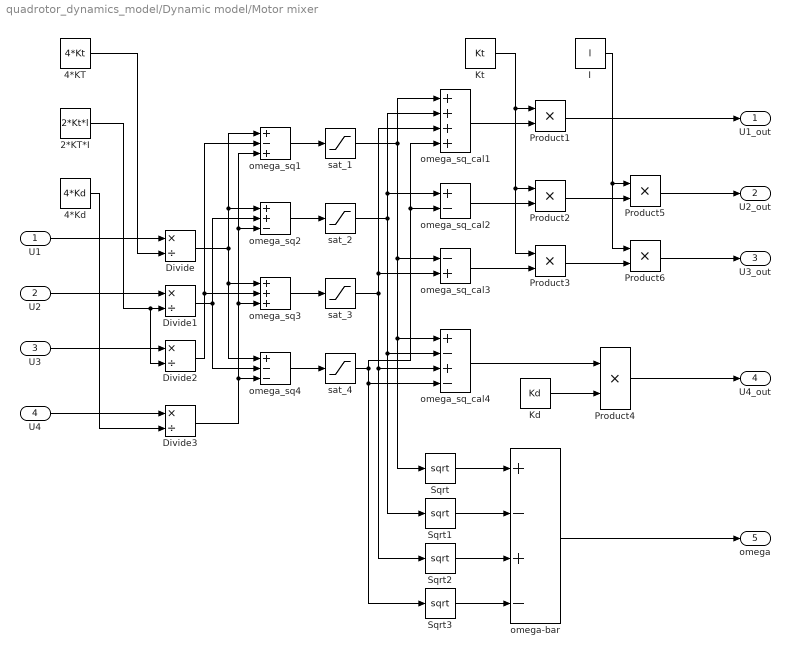
== system quadrotor_dynamics_model/Dynamic model/Motor mixer ==
  U1 : Inport
  U2 : Inport  Port=2
  U3 : Inport  Port=3
  U4 : Inport  Port=4
  2*KT*I : Constant  Value=2*Kt*l
  4*KT : Constant  Value=4*Kt
  4*Kd : Constant  Value=4*Kd
  Divide{,1..3} (4 alike) : Product  Inputs=*/
  I : Constant  Value=l
  Kd : Constant  Value=Kd
  Kt : Constant  Value=Kt
  Product{1..6} (6 alike) : Product
  Sqrt{,1..3} (4 alike) : Sqrt  OutputSignalType=real
  omega-bar : Sum  Inputs=+-+-
  omega_sq1 : Sum  Inputs=+-+
  omega_sq2 : Sum  Inputs=++-
  omega_sq3 : Sum  Inputs=+++
  omega_sq4 : Sum  Inputs=+--
  omega_sq_cal1 : Sum  Inputs=++++
  omega_sq_cal2 : Sum  Inputs=+-
  omega_sq_cal3 : Sum  Inputs=-+
  omega_sq_cal4 : Sum  Inputs=+-+-
  sat_1 : Saturate  UpperLimit=omega_sq_max  LowerLimit=0  ZeroCross=off
  sat_2 : Saturate  UpperLimit=omega_sq_max  LowerLimit=0  LinearizeAsGain=off  ZeroCross=off
  sat_3 : Saturate  UpperLimit=omega_sq_max  LowerLimit=0  ZeroCross=off
  sat_4 : Saturate  UpperLimit=omega_sq_max  LowerLimit=0  ZeroCross=off
  U1_out : Outport
  U2_out : Outport  Port=2
  U3_out : Outport  Port=3
  U4_out : Outport  Port=4
  omega : Outport  Port=5
  wires:
  U1/1 -> Divide/1
  U2/1 -> Divide1/1
  U3/1 -> Divide2/1
  U4/1 -> Divide3/1
  4*KT/1 -> Divide/2
  2*KT*I/1 -> Divide2/2, Divide1/2
  4*Kd/1 -> Divide3/2
  Divide/1 -> omega_sq4/1, omega_sq3/1, omega_sq2/1, omega_sq1/1
  Divide1/1 -> omega_sq4/2, omega_sq2/2
  Divide2/1 -> omega_sq3/2, omega_sq1/2
  Divide3/1 -> omega_sq1/3, omega_sq2/3, omega_sq3/3, omega_sq4/3
  omega_sq1/1 -> sat_1/1
  omega_sq2/1 -> sat_2/1
  omega_sq3/1 -> sat_3/1
  omega_sq4/1 -> sat_4/1
  omega-bar/1 -> omega/1
  Kt/1 -> Product3/1, Product2/1, Product1/1
  omega_sq_cal1/1 -> Product1/2
  omega_sq_cal2/1 -> Product2/2
  omega_sq_cal3/1 -> Product3/2
  I/1 -> Product6/1, Product5/1
  Product3/1 -> Product6/2
  Product2/1 -> Product5/2
  omega_sq_cal4/1 -> Product4/1
  Kd/1 -> Product4/2
  Product1/1 -> U1_out/1
  Product5/1 -> U2_out/1
  Product6/1 -> U3_out/1
  Product4/1 -> U4_out/1
  sat_1/1 -> omega_sq_cal1/1, omega_sq_cal3/1, omega_sq_cal4/1, Sqrt/1
  sat_2/1 -> omega_sq_cal2/1, omega_sq_cal1/2, omega_sq_cal4/2, Sqrt1/1
  sat_3/1 -> omega_sq_cal3/2, omega_sq_cal1/3, omega_sq_cal4/3, Sqrt2/1
  sat_4/1 -> omega_sq_cal1/4, omega_sq_cal2/2, omega_sq_cal4/4, Sqrt3/1
  Sqrt/1 -> omega-bar/1
  Sqrt1/1 -> omega-bar/2
  Sqrt2/1 -> omega-bar/3
  Sqrt3/1 -> omega-bar/4

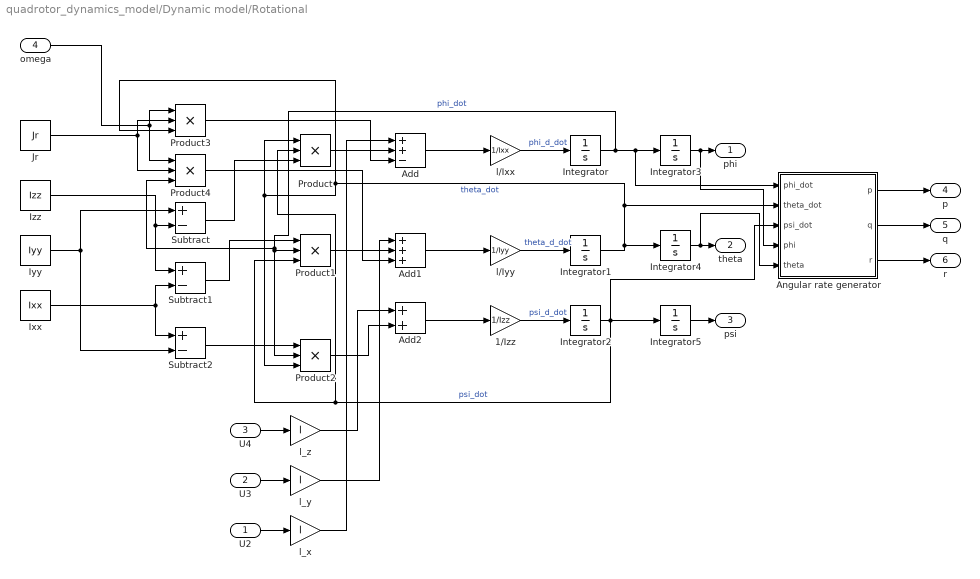
== system quadrotor_dynamics_model/Dynamic model/Rotational ==
  U2 : Inport
  U3 : Inport  Port=2
  U4 : Inport  Port=3
  omega : Inport  Port=4
  1/Izz : Gain  Gain=1/Izz
  Add : Sum  Inputs=++-
  Add1 : Sum  Inputs=+++
  Add2 : Sum
  Angular rate generator : Subsystem
  Integrator : Integrator  InitialCondition=rpy_dot_in(1)  ZeroCross=off
  Integrator1 : Integrator  InitialCondition=rpy_dot_in(2)  ZeroCross=off
  Integrator2 : Integrator  InitialCondition=rpy_dot_in(3)  ZeroCross=off
  Integrator3 : Integrator  InitialCondition=rpy_in(1)  ZeroCross=off
  Integrator4 : Integrator  InitialCondition=rpy_in(2)  UpperSaturationLimit=0.1745  LowerSaturationLimit=-0.1745  ZeroCross=off
  Integrator5 : Integrator  InitialCondition=rpy_in(3)  UpperSaturationLimit=3.1416  LowerSaturationLimit=-3.1416  ZeroCross=off
  Ixx : Constant  Value=Ixx
  Iyy : Constant  Value=Iyy
  Izz : Constant  Value=Izz
  Jr : Constant  Value=Jr
  Product{,1..4} (5 alike) : Product  Inputs=3
  Subtract : Sum  Inputs=+-
  Subtract1 : Sum  Inputs=+-
  Subtract2 : Sum  Inputs=+-
  l/Ixx : Gain  Gain=1/Ixx
  l/Iyy : Gain  Gain=1/Iyy
  l_x : Gain  Gain=l
  l_y : Gain  Gain=l
  l_z : Gain  Gain=l
  phi : Outport
  theta : Outport  Port=2
  psi : Outport  Port=3
  p : Outport  Port=4
  q : Outport  Port=5
  r : Outport  Port=6
  wires:
  l/Ixx/1 -> Integrator/1  "phi_d_dot"
  Integrator/1 -> Product1/2, Product2/2, Product4/3, Angular rate generator/1(phi_dot), Integrator3/1  "phi_dot"
  Integrator1/1 -> Angular rate generator/2(theta_dot), Product3/3, Product2/3, Product/1, Integrator4/1  "theta_dot"
  l/Iyy/1 -> Integrator1/1  "theta_d_dot"
  1/Izz/1 -> Integrator2/1  "psi_d_dot"
  Integrator2/1 -> Integrator5/1, Angular rate generator/3(psi_dot), Product1/3, Product/2  "psi_dot"
  Integrator3/1 -> Angular rate generator/4(phi), phi/1
  Integrator4/1 -> theta/1, Angular rate generator/5(theta)
  Integrator5/1 -> psi/1
  U2/1 -> l_x/1
  l_x/1 -> Add/1
  l_y/1 -> Add1/1
  U3/1 -> l_y/1
  l_z/1 -> Add2/1
  U4/1 -> l_z/1
  Iyy/1 -> Subtract2/2, Subtract/1
  Izz/1 -> Subtract1/1, Subtract/2
  Subtract/1 -> Product/3
  Ixx/1 -> Subtract1/2, Subtract2/1
  Subtract1/1 -> Product1/1
  Product/1 -> Add/2
  Add/1 -> l/Ixx/1
  Product1/1 -> Add1/2
  Add1/1 -> l/Iyy/1
  Subtract2/1 -> Product2/1
  Product2/1 -> Add2/2
  Add2/1 -> 1/Izz/1
  Jr/1 -> Product3/2, Product4/2
  Angular rate generator/1(p) -> p/1
  Angular rate generator/2(q) -> q/1
  Angular rate generator/3(r) -> r/1
  omega/1 -> Product3/1, Product4/1
  Product3/1 -> Add/3
  Product4/1 -> Add1/3

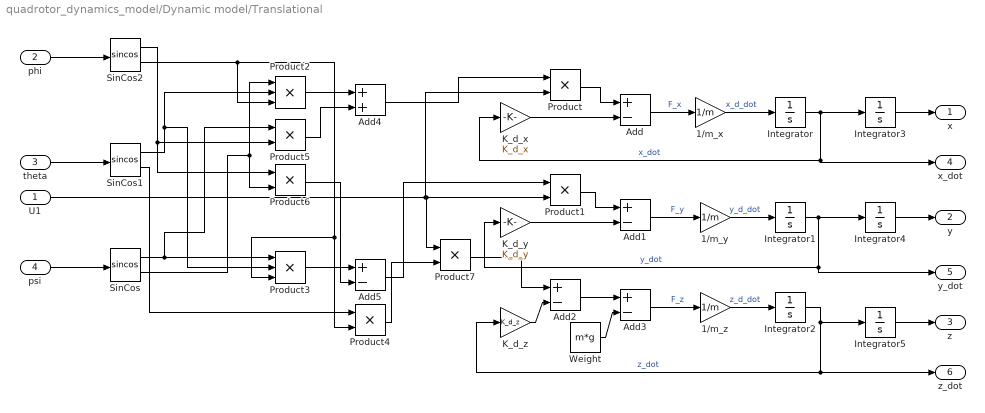
== system quadrotor_dynamics_model/Dynamic model/Translational  ==
  U1 : Inport
  phi : Inport  Port=2
  theta : Inport  Port=3
  psi : Inport  Port=4
  1/m_x : Gain  Gain=1/m
  1/m_y : Gain  Gain=1/m
  1/m_z : Gain  Gain=1/m
  Add{,1..3,5} (5 alike) : Sum  Inputs=+-
  Add4 : Sum
  Integrator : Integrator  InitialCondition=xyz_dot_in(1)  ZeroCross=off
  Integrator1 : Integrator  InitialCondition=xyz_dot_in(2)  ZeroCross=off
  Integrator2 : Integrator  InitialCondition=xyz_dot_in(3)  ZeroCross=off
  Integrator3 : Integrator  InitialCondition=xyz_in(1)  ZeroCross=off
  Integrator4 : Integrator  InitialCondition=xyz_in(2)  ZeroCross=off
  Integrator5 : Integrator  InitialCondition=xyz_in(3)  ZeroCross=off
  K_d_x : Gain  Gain=K_d_x
  K_d_y : Gain  Gain=K_d_y
  K_d_z : Gain  Gain=K_d_z
  Product{,1,4..7} (6 alike) : Product
  Product2 : Product  Inputs=3
  Product3 : Product  Inputs=3
  SinCos : Trigonometry  Operator=sincos
  SinCos1 : Trigonometry  Operator=sincos
  SinCos2 : Trigonometry  Operator=sincos
  Weight : Constant  Value=m*g
  x : Outport
  y : Outport  Port=2
  z : Outport  Port=3
  x_dot : Outport  Port=4
  y_dot : Outport  Port=5
  z_dot : Outport  Port=6
  wires:
  Integrator2/1 -> K_d_z/1, z_dot/1, Integrator5/1  "z_dot"
  U1/1 -> Product/2, Product7/1, Product1/2
  K_d_z/1 -> Add2/2
  Product/1 -> Add/1
  Integrator5/1 -> z/1
  Integrator1/1 -> y_dot/1, K_d_y/1, Integrator4/1  "y_dot"
  K_d_y/1 -> Add1/2
  Add2/1 -> Add3/1
  Add/1 -> 1/m_x/1  "F_x"
  K_d_x/1 -> Add/2
  Add3/1 -> 1/m_z/1  "F_z"
  Add5/1 -> Product1/1
  Product1/1 -> Add1/1
  Integrator/1 -> Integrator3/1, x_dot/1, K_d_x/1  "x_dot"
  Add1/1 -> 1/m_y/1  "F_y"
  Integrator4/1 -> y/1
  Integrator3/1 -> x/1
  Weight/1 -> Add3/2
  1/m_x/1 -> Integrator/1  "x_d_dot"
  1/m_y/1 -> Integrator1/1  "y_d_dot"
  1/m_z/1 -> Integrator2/1  "z_d_dot"
  SinCos/2 -> Product6/2, Product2/1
  SinCos1/1 -> Product3/2, Product2/2
  SinCos2/2 -> Product4/2, Product3/3, Product2/3
  Product2/1 -> Add4/1
  SinCos/1 -> Product5/1, Product3/1
  SinCos2/1 -> Product6/1, Product5/2
  Product5/1 -> Add4/2
  Add4/1 -> Product/1
  Product3/1 -> Add5/1
  Product6/1 -> Add5/2
  Product7/1 -> Add2/1
  SinCos1/2 -> Product4/1
  Product4/1 -> Product7/2
  psi/1 -> SinCos/1
  theta/1 -> SinCos1/1
  phi/1 -> SinCos2/1

== system quadrotor_dynamics_model/Dynamic model/Rotational/Angular rate generator ==
  phi_dot : Inport
  theta_dot : Inport  Port=2
  psi_dot : Inport  Port=3
  phi : Inport  Port=4
  theta : Inport  Port=5
  Subsystem : Subsystem
  "p " : Subsystem
  "q " : Subsystem
  q 1 : Subsystem
  p : Outport
  q : Outport  Port=2
  r : Outport  Port=3
  wires:
  psi_dot/1 -> q 1/1(psi_dot), "q "/1(psi_dot), "p "/3(psi_dot)
  phi_dot/1 -> "p "/1(phi_dot)
  "p "/1(p) -> p/1
  theta_dot/1 -> q 1/2(theta_dot), "q "/2(theta_dot)
  "q "/1(q) -> q/1
  phi/1 -> Subsystem/1(phi)
  theta/1 -> Subsystem/2(theta)
  Subsystem/1(sin theta) -> "p "/2(sin theta)
  Subsystem/2(cos phi) -> q 1/3(cos phi), "q "/3(cos phi)
  Subsystem/3(sin phi) -> q 1/4(sin phi), "q "/4(sin phi)
  Subsystem/4(cos theta) -> q 1/5(cos theta), "q "/5(cos theta)
  q 1/1(r) -> r/1

== system quadrotor_dynamics_model/Dynamic model/Rotational/Angular rate generator/Subsystem ==
  phi : Inport
  theta : Inport  Port=2
  Cos : Trigonometry  Operator=cos
  Cos1 : Trigonometry  Operator=cos
  Sin : Trigonometry
  Sin1 : Trigonometry
  sin theta : Outport
  cos phi : Outport  Port=2
  sin phi : Outport  Port=3
  cos theta : Outport  Port=4
  wires:
  Sin1/1 -> sin phi/1
  phi/1 -> Sin1/1, Cos/1
  Sin/1 -> sin theta/1
  Cos1/1 -> cos theta/1
  Cos/1 -> cos phi/1
  theta/1 -> Cos1/1, Sin/1

== system quadrotor_dynamics_model/Dynamic model/Rotational/Angular rate generator/p  ==
  phi_dot : Inport
  sin theta : Inport  Port=2
  psi_dot : Inport  Port=3
  Add : Sum  Inputs=+-
  Product : Product
  p : Outport
  wires:
  Product/1 -> Add/2
  sin theta/1 -> Product/2
  Add/1 -> p/1
  phi_dot/1 -> Add/1
  psi_dot/1 -> Product/1

== system quadrotor_dynamics_model/Dynamic model/Rotational/Angular rate generator/q  ==
  psi_dot : Inport
  theta_dot : Inport  Port=2
  cos phi : Inport  Port=3
  sin phi : Inport  Port=4
  cos theta : Inport  Port=5
  Add1 : Sum
  Product1 : Product
  Product2 : Product  Inputs=3
  q : Outport
  wires:
  Product2/1 -> Add1/2
  sin phi/1 -> Product2/2
  psi_dot/1 -> Product2/1
  cos theta/1 -> Product2/3
  Add1/1 -> q/1
  Product1/1 -> Add1/1
  theta_dot/1 -> Product1/2
  cos phi/1 -> Product1/1

== system quadrotor_dynamics_model/Dynamic model/Rotational/Angular rate generator/q 1 ==
  psi_dot : Inport
  theta_dot : Inport  Port=2
  cos phi : Inport  Port=3
  sin phi : Inport  Port=4
  cos theta : Inport  Port=5
  Add1 : Sum  Inputs=-+
  Product1 : Product
  Product2 : Product  Inputs=3
  r : Outport
  wires:
  Product2/1 -> Add1/2
  psi_dot/1 -> Product2/1
  cos theta/1 -> Product2/3
  Add1/1 -> r/1
  Product1/1 -> Add1/1
  theta_dot/1 -> Product1/2
  sin phi/1 -> Product1/1
  cos phi/1 -> Product2/2
